simulink model "W06_C_square"  (R2024b)
settings: Solver=ode4  StartTime=0  StopTime=T_final  FixedStep=h  RelTol=1e-3
values from neighbouring files (symbols this model uses):
  beta_c = 0    [W06_0_setup.m]
  k_neg = cfg.k_neg    [W06_0_setup.m]
  k_pos = cfg.k_pos    [W06_0_setup.m]
  mp = 25    [W06_0_setup.m]
  N_big = 50    [W06_0_setup.m]
  N_cmd = 20    [W06_0_setup.m]
  rp = [0.05 0 -0.35]'    [W06_0_setup.m]
  use_kneg = 1    [W06_0_setup.m]
  V_c = 0    [W06_0_setup.m]
  x0 = zeros(12,1)    [W06_0_setup.m]
  X_big = 220    [W06_0_setup.m]
  X_cmd = 100    [W06_0_setup.m]
  Y_cmd = 30    [W06_0_setup.m]
  y_pont = cfg.y_pont    [W06_0_setup.m]
settings Model: Creator=admin  LastModifiedBy=admin
settings DataIOCC: ReturnWorkspaceOutputs=off

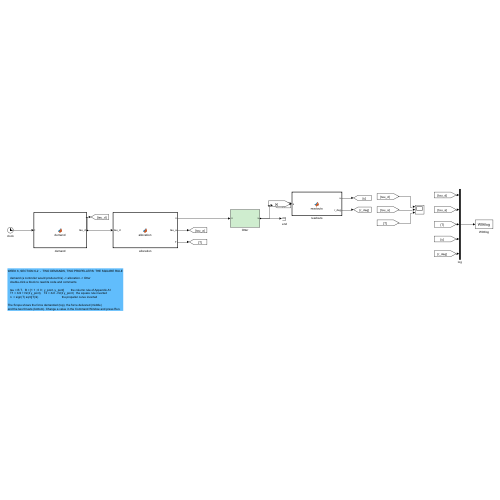
[thumbnail: Simulink's stored preview of the top-level diagram]
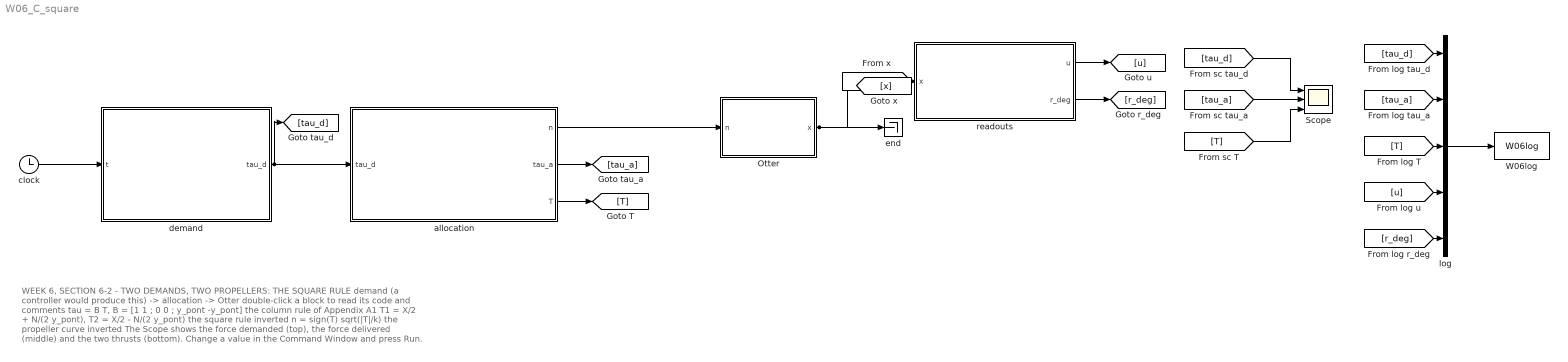
== system W06_C_square ==
  note: WEEK 6, SECTION 6-2  -  TWO DEMANDS, TWO PROPELLERS: THE SQUARE RULE
      |
      |    demand (a controller would produce this) -> allocation -> Otter
      |    double-click a block to read its code and comments
      |
      |    tau = B T,   B = [1 1 ; 0 0 ; y_pont -y_pont]        the column rule of Appendix A1
      |    T1 = X/2 + N/(2 y_pont),   T2 = X/2 - N/(2 y_pont)   the square rule inverted
      |    n  = sign(T) sqrt(|T|/k)                             the propeller curve inverted
      |
      | The Scope shows the force demanded (top), the force delivered (middle)
      | and the two thrusts (bottom). Change a value in the Command Window and press Run.
  Otter : Subsystem
  Scope : Scope  NumInputPorts=3
  W06log : ToWorkspace  VariableName=W06log  SaveFormat=Structure With Time  SampleTime=-1
  allocation : MATLAB Function  TreatAsAtomicUnit=on
  clock : Clock
  demand : MATLAB Function  TreatAsAtomicUnit=on
  end : Terminator
  log : Mux  Inputs=5
  readouts : MATLAB Function  TreatAsAtomicUnit=on
  wires:
  clock/1 -> demand/1(t)
  demand/1(tau_d) -> [tau_d], allocation/1(tau_d)
  allocation/2(tau_a) -> [tau_a]
  allocation/3(T) -> [T]
  allocation/1(n) -> Otter/1(n)
  Otter/1(x) -> [x], end/1
  [x] -> readouts/1(x)
  readouts/1(u) -> [u]
  readouts/2(r_deg) -> [r_deg]
  [tau_d] -> Scope/1
  [tau_a] -> Scope/2
  [T] -> Scope/3
  [tau_d] -> log/1
  [tau_a] -> log/2
  [T] -> log/3
  [u] -> log/4
  [r_deg] -> log/5
  log/1 -> W06log/1

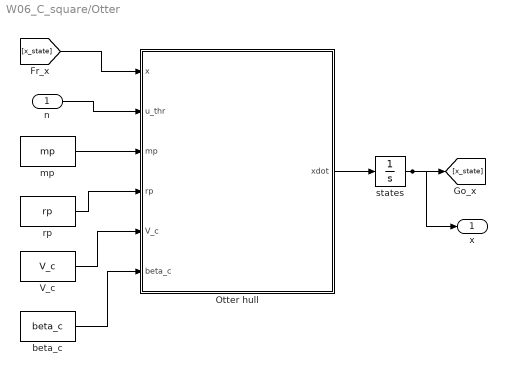
== system W06_C_square/Otter ==
  n : Inport
  Otter hull : MATLAB Function  TreatAsAtomicUnit=on
  V_c : Constant  Value=V_c
  beta_c : Constant  Value=beta_c
  mp : Constant  Value=mp
  rp : Constant  Value=rp
  states : Integrator  InitialCondition=x0
  x : Outport
  wires:
  [x_state] -> Otter hull/1(x)
  V_c/1 -> Otter hull/5(V_c)
  n/1 -> Otter hull/2(u_thr)
  states/1 -> [x_state], x/1
  Otter hull/1(xdot) -> states/1
  beta_c/1 -> Otter hull/6(beta_c)
  mp/1 -> Otter hull/3(mp)
  rp/1 -> Otter hull/4(rp)

== matlab function W06_C_square/allocation ==
  data: tau_d input; n output double size=[2 1]; tau_a output; T output; y_pont parameter; k_pos parameter; k_neg parameter; use_kneg parameter
function [n, tau_a, T] = allocation(tau_d, y_pont, k_pos, k_neg, use_kneg)
%#codegen
%  ────────────────────────────────────────────────────────────────────────
%  1) 일반화 힘 -> 추력 둘 / from the demanded force to two thrusts
%
%     이 선체의 제어 유효행렬은 (부록 A1 의 열 규칙에서)
%     The control effectiveness matrix of this hull, from the column rule of A1:
%
%         tau = B T,   B = [ 1        1      ;
%                            0        0      ;
%                            y_pont  -y_pont ]
%
%     B 의 둘째 행이 0 이다 — 두 추진기 모두 옆으로 밀지 못한다. 그래서 Y 는
%     어떤 T 로도 만들 수 없고, 최소자승해는 그것을 조용히 버린다 (§6-3).
%     The second row is zero: neither propeller pushes sideways, so no T can
%     produce Y, and the least-squares solution simply drops it (§6-3).
%
%     남은 두 행은 정사각이고 가역이다 / the remaining two rows are square and invertible:
%
%         T1 = X/2 + N/(2 y_pont),   T2 = X/2 - N/(2 y_pont)
T1 = tau_d(1)/2 + tau_d(3)/(2*y_pont);
T2 = tau_d(1)/2 - tau_d(3)/(2*y_pont);
%  ────────────────────────────────────────────────────────────────────────
%  3) 추력 -> 회전수 / thrust to shaft speed
%     프로펠러 곡선은 T = k n|n| 이고, k 가 전진과 후진에서 다르다 (1주차).
%     따라서 역함수도 방향에 따라 다른 k 를 써야 한다 — use_kneg = 0 으로 두면
%     후진에도 k_pos 를 써서 요구보다 적은 힘이 나온다 (§6-5).
%     The propeller curve is T = k n|n| with a different k astern (Week 1), so
%     the inverse must use the same k. With use_kneg = 0 it uses k_pos both
%     ways, and the vessel gets less than it asked for going astern.
k1 = k_pos;  if T1 < 0 && use_kneg == 1, k1 = k_neg; end
k2 = k_pos;  if T2 < 0 && use_kneg == 1, k2 = k_neg; end
n = [sign(T1)*sqrt(abs(T1)/k1); sign(T2)*sqrt(abs(T2)/k2)];
%  ────────────────────────────────────────────────────────────────────────
%  4) 실제로 전달된 힘 / the force actually delivered
%     축이 그 회전수로 돌 때 프로펠러가 내는 추력을 다시 곡선으로 계산하고,
%     그것을 B 로 곱한다. 요구와 다르면 그 차이가 이 주차의 관찰 대상이다.
%     The thrust those shafts really produce, put back through B. Any gap
%     between this and the demand is what this week is about.
T1a = k_pos*n(1)*abs(n(1));  if n(1) < 0, T1a = k_neg*n(1)*abs(n(1)); end
T2a = k_pos*n(2)*abs(n(2));  if n(2) < 0, T2a = k_neg*n(2)*abs(n(2)); end
tau_a = [T1a + T2a; 0; y_pont*(T1a - T2a)];
T = [T1a; T2a];

== matlab function W06_C_square/demand ==
  data: t input; tau_d output double size=[3 1]; X_cmd parameter; Y_cmd parameter; N_cmd parameter; X_big parameter; N_big parameter
function tau_d = demand(t, X_cmd, Y_cmd, N_cmd, X_big, N_big)
%#codegen
%  이 블록은 제어기를 대신한다. 3~5주차에서는 속도·선수각 제어기가 이 세 수를 냈다.
%  이번 주가 묻는 것은 그 다음이다: 이 요구를 추진기 둘에 어떻게 나누는가?
%  This block stands in for the controllers of Weeks 3 to 5, which produced
%  these three numbers. This week asks what happens next: how are they shared
%  between two propellers?
%
%     tau_d = [X ; Y ; N]   전진력 [N], 횡력 [N], 요 모멘트 [N m]
tau_d = [0; 0; 0];
%  6-2 의 시간표: 전진력만, 그 다음 요 모멘트를 좌우로 / surge alone, then yaw both ways
if     t >=  5 && t < 15, tau_d = [X_cmd; 0;  0    ];
elseif t >= 15 && t < 25, tau_d = [X_cmd; 0;  N_cmd];
elseif t >= 25 && t < 35, tau_d = [X_cmd; 0; -N_cmd];
end

== matlab function W06_C_square/Otter/Otter hull ==
  data: x input; xdot output double size=[12 1]; u_thr input; mp input; rp input; V_c input; beta_c input
function xdot = otter_hull(x, u_thr, mp, rp, V_c, beta_c)
% Fossen's otter.m, called unchanged from Tools/MSS/VESSELS.
%
%   x       12 states, fed back from the integrator
%   u_thr   propeller shaft speeds [rad/s]
%
% otter.m is not written for code generation, so the call is extrinsic and
% xdot has to be pre-sized for Simulink to know the output width.
coder.extrinsic('otter');

xdot = zeros(12,1);
xdot = otter(x, u_thr, mp, rp, V_c, beta_c);
end

== matlab function W06_C_square/readouts ==
  data: x input; u output double size=[1 1]; r_deg output
function [u, r_deg] = readouts(x)
%#codegen
%  상태에서 보고 싶은 둘만 꺼낸다 / the two states this week watches
%     x = [u v w p q r  N E z  phi theta psi]
u     = x(1);           % 전진속도 / surge speed   [m/s]
r_deg = x(6)*180/pi;    % 회두율 / yaw rate        [deg/s]
